simulink model "DirectedEvent6"  (R2020b)
settings: Solver=VariableStepAuto  StartTime=0.0  StopTime=0.1  RelTol=1e-3
settings Model: Creator=86188  LastModifiedBy=apple
settings DataIOCC: ReturnWorkspaceOutputs=off
settings DebuggingCC: ArithmeticOperatorsInVariantConditions=warning
settings SFSimCC: SimUseLocalCustomCode=off  CustomCodeUndefinedFunction=UseInterfaceOnly
settings RTWCC: RTWUseLocalCustomCode=off

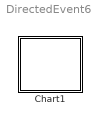
== system DirectedEvent6 ==
  Chart1 : Stateflow chart  TreatAsAtomicUnit=on

== stateflow chart DirectedEvent6/Chart1 ==
  settings: updateMethod=DISCRETE  sampleTime=0.1
  state A
  state B
  state C
    state C1
    state C2
    (default) -> C1
    C1 -> C2 : F{fprintf("d")}
  (default) -> A : {data = 1;}
  A -> B [order 1] : [data==1]{data=2;fprintf("a");send(F,A);fprintf("b")}
  A -> C [order 2] : F{fprintf("c")}
  data: data local =1
  events: F local FUNCTION_CALL_EVENT
